simulink model "Heading_Mode"  (R2013a)
settings: configuration reference "DO178ConfigSet" (kept outside this file)
model workspace (MAT data in the model file):
  hdgGain = Simulink.Parameter
  hdgGain.Value = 0.015
  hdgGain.DataType = 'auto'
  hdgGain.Min = 0
libraries: AP_Lib x1, simulink x1
settings Model: RequirementInfo={} %GIDa_fe9045fd_0412_4b6e_8206_617cc20e6fde  CovSaveName=covdata_rollAP  CovMetricSettings=dcmtrwe  CovHTMLOptions=-aTS=1 -bRG=1 -bTC=1 -hTR=1 -nFC=0 -scm=1 -bcm=1  CovHtmlReporting=off  CovCumulativeVarName=covCumulativeData_rollAP  CovCumulativeReport=on  CovReportOnPause=off  CovModelRefEnable=off  Creator=bpotter  LastModifiedBy=syoon

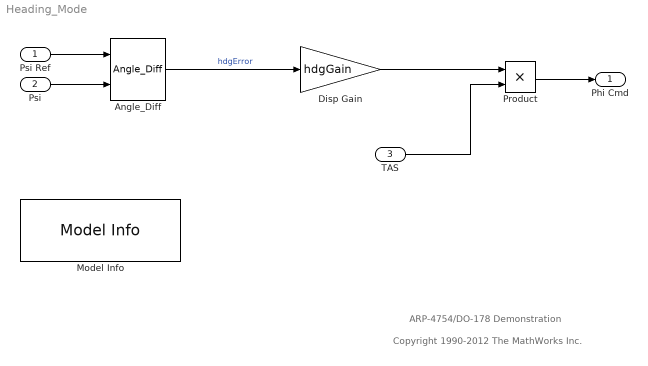
== system Heading_Mode ==
  note: Copyright 1990-2012 The MathWorks Inc.
  note: ARP-4754/DO-178 Demonstration
  Psi Ref : Inport  RequirementInfo={'other' '..\requirements\do178b_autopilot_requirements.docx' '@Simulink_requirement_item_10' 'true' '1.10. Heading Performance' '' } %GIDa_7dc03c75_5e34_4e08_bb6f_6d840def0f56  OutDataTypeStr=double  PortDimensions=1  SampleTime=1/40  Interpolate=off
  Psi : Inport  RequirementInfo={'other' '..\requirements\do178b_autopilot_requirements.docx' '@Simulink_requirement_item_10' 'true' '1.10. Heading Performance' '' } %GIDa_4169e82d_42c5_44c7_a191_9b5ca9dcb70a  Port=2  OutDataTypeStr=double  PortDimensions=1  SampleTime=1/40  Interpolate=off
  TAS : Inport  RequirementInfo={'other' '..\requirements\do178b_autopilot_requirements.docx' '@Simulink_requirement_item_10' 'true' '1.10. Heading Performance' '' } %GIDa_f893e673_5937_4a6a_88ec_5c2959f3360e  Port=3  OutDataTypeStr=double  PortDimensions=1  SampleTime=1/40  Interpolate=off
  Angle_Diff : AP_Lib/Angle_Diff  RequirementInfo={'other' '..\requirements\do178b_autopilot_requirements.docx' '@Simulink_requirement_item_10' 'true' '1.10. Heading Performance' '' } %GIDa_e9ab25ca_e212_4420_986d_476c64d5e13d
      settings: AttributesFormatString=-180 deg to +180 deg range
  Disp Gain : Gain  RequirementInfo={'other' '..\requirements\do178b_autopilot_requirements.docx' '@Simulink_requirement_item_10' 'true' '1.10. Heading Performance' '' } %GIDa_e43ec5f2_7e00_48d9_b3be_d6b2fb8df9a5  Gain=hdgGain
  Model Info : simulink/Model-Wide Utilities/Model Info  InitialBlockCM=None  BlockCM=None  Frame=on  DisplayStringWithTags=|  HorizontalTextAlignment=Left  LeftAlignmentValue=0.02  SourceBlockDiagram=Heading_Mode  TagMaxNumber=20
      | Heading Mode
      | Author: %<LastModifiedBy>
      | Version: %<ModelVersion>
      | Date: %<LastModificationDate>
  Product : Product  RequirementInfo={'other' '..\requirements\do178b_autopilot_requirements.docx' '@Simulink_requirement_item_10' 'true' '1.10. Heading Performance' '' } %GIDa_ab0fdff5_b5b7_4090_bee6_e4de829092e0  RndMeth=Zero
  Phi Cmd : Outport  RequirementInfo={'other' '..\requirements\do178b_autopilot_requirements.docx' '@Simulink_requirement_item_10' 'true' '1.10. Heading Performance' '' } %GIDa_b1e9aa33_d2c6_47b6_aeae_2214d48474ed  OutDataTypeStr=double  PortDimensions=1  SampleTime=1/40
  wires:
  Product/1 -> Phi Cmd/1
  Disp Gain/1 -> Product/1
  Angle_Diff/1 -> Disp Gain/1  "hdgError"
  Psi Ref/1 -> Angle_Diff/1
  TAS/1 -> Product/2
  Psi/1 -> Angle_Diff/2
